simulink model "modelSimpleGenset"  (R2019a)
settings: Solver=FixedStepAuto  StartTime=0.0  StopTime=10.0  FixedStep=1e-1  RelTol=1e-3
model workspace (MAT data in the model file):
  avrDroop = 0.01
  avrKI = 10
  avrKP = 40
  governorDroop = 0.02
  inductiveInnerResistance = 0.48
  initialFieldVoltage = 0.676611722086
  maxFieldVoltage = 20
  minFieldVoltage = 0.01
  noLoadFrequency = 1.0101010101
  ratedPower = 9100000
  resistiveInnerResistance = 0.0019
values from neighbouring files (symbols this model uses):
  numberOfBuses = 2    [init.m]
libraries: simulink x8
settings Model: DataDictionary=dataGenerator.sldd  ParameterArgumentNames=ratedPower  OrderedModelArguments=off  Creator=michel.miyazaki  LastModifiedBy=thomas.evang
settings SimscapeCC: EditingMode=Restricted

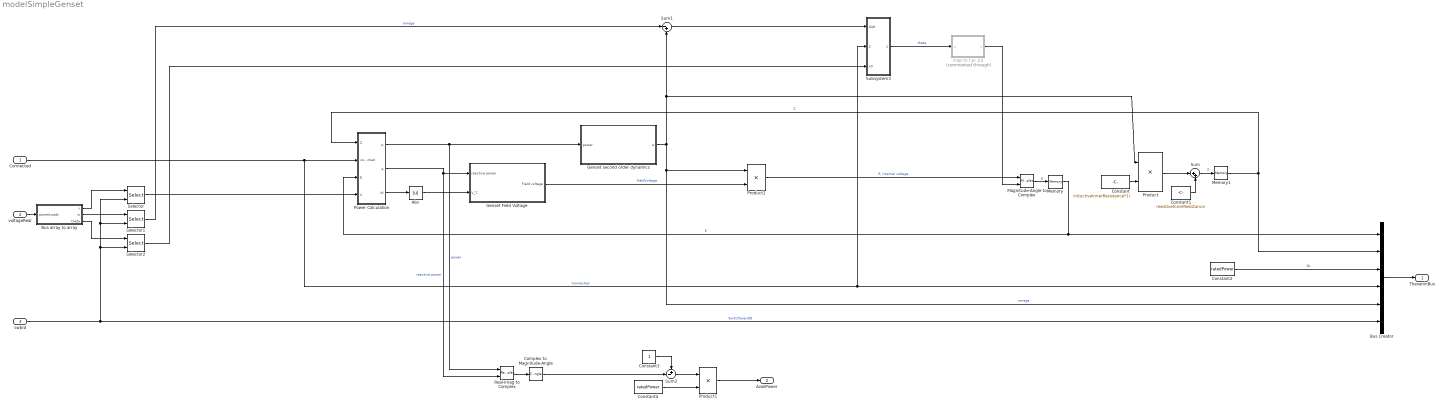
== system modelSimpleGenset ==
  Connected : Inport  OutDataTypeStr=boolean
  voltageReal : Inport  Port=2  OutDataTypeStr=Bus: swb  PortDimensions=[1 numberOfBuses]  Interpolate=off  BusOutputAsStruct=on
  swbId : Inport  Port=3
  Abs : Abs
  Bus Creator : BusCreator  Inputs=6  OutDataTypeStr=Bus: TheveninBus
  Bus array to array : Subsystem  TreatAsAtomicUnit=on
  Complex to Magnitude-Angle : ComplexToMagnitudeAngle  Output=Magnitude
  Constant : Constant  Value=inductiveInnerResistance*1i
  Constant1 : Constant  Value=resistiveInnerResistance
  Constant2 : Constant  Value=ratedPower
  Constant3 : Constant
  Constant4 : Constant  Value=ratedPower
  Genset Field Voltage : Subsystem
  Genset second order dynamics : Subsystem
  Magnitude-Angle to Complex : MagnitudeAngleToComplex
  Memory : Memory  InitialCondition=0.43*(1+1*1i)  LinearizeMemory=on  LinearizeAsDelay=on
  Memory1 : Memory  InitialCondition=resistiveInnerResistance+inductiveInnerResistance*1i*noLoadFrequency  LinearizeMemory=on  LinearizeAsDelay=on
  Power Calculation : Subsystem
  Product : Product
  Product1 : Product  Inputs=**  RndMeth=Zero
  Product2 : Product  Inputs=**  RndMeth=Zero
  Real-Imag to Complex : RealImagToComplex
  Selector : Selector  IndexOptions=Index vector (port)  Indices=[1 3]  OutputSizes=1
  Selector1 : Selector  IndexOptions=Index vector (port)  Indices=[1 3]  OutputSizes=1
  Selector2 : Selector  IndexOptions=Index vector (port)  Indices=[1 3]  OutputSizes=1
  Subsystem3 : Subsystem
  Sum : Sum  Inputs=|++
  Sum1 : Sum  Inputs=|-+
  Sum2 : Sum  Inputs=+-|
  "map to [-pi, pi]" : Subsystem  Commented=through
  TheveninBus : Outport  OutDataTypeStr=Bus: TheveninBus  BusOutputAsStruct=on
  AvailPower : Outport  Port=2  BusOutputAsStruct=on
  wires:
  Constant/1 -> Product/2
  Selector1/1 -> Sum1/1  "omega"
  Selector2/1 -> Subsystem3/3(x0)
  Product/1 -> Sum/1
  Constant1/1 -> Sum/2
  Sum/1 -> Memory1/1  "Z"
  Connected/1 -> Power Calculation/2(connected), Subsystem3/2(reset), Bus Creator/4  "Connected"
  Magnitude-Angle to Complex/1 -> Memory/1  "E"
  Sum1/1 -> Subsystem3/1(d/dt)
  Subsystem3/1(Out1) -> "map to [-pi, pi]"/1(u)  "theta"
  Product2/1 -> Magnitude-Angle to Complex/1  "E, internal voltage"
  Power Calculation/2(q) -> Real-Imag to Complex/2, Genset Field Voltage/1(reactive power)  "reactive power"
  Genset Field Voltage/1(Field voltage) -> Product2/2  "fieldVoltage"
  Power Calculation/1(p) -> Genset second order dynamics/1(power), Real-Imag to Complex/1  "power"
  Power Calculation/3(Vt) -> Abs/1
  Abs/1 -> Genset Field Voltage/2(V_T)
  Genset second order dynamics/1(w) -> Bus Creator/5, Product2/1, Product/1, Sum1/2  "omega"
  Memory1/1 -> Bus Creator/2, Power Calculation/1(Z)  "Z"
  Memory/1 -> Bus Creator/1, Power Calculation/3(E)  "E"
  "map to [-pi, pi]"/1(y) -> Magnitude-Angle to Complex/2
  Selector/1 -> Power Calculation/4(V)
  voltageReal/1 -> Bus array to array/1(powerLoads)
  Bus Creator/1 -> TheveninBus/1
  Constant2/1 -> Bus Creator/3  "Sb"
  swbId/1 -> Selector2/2, Selector1/2, Selector/2, Bus Creator/6  "SwitchboardID"
  Bus array to array/2(w) -> Selector1/1
  Bus array to array/3(theta) -> Selector2/1
  Bus array to array/1(v) -> Selector/1
  Sum2/1 -> Product1/1
  Real-Imag to Complex/1 -> Complex to Magnitude-Angle/1
  Constant4/1 -> Product1/2
  Complex to Magnitude-Angle/1 -> Sum2/2
  Constant3/1 -> Sum2/1
  Product1/1 -> AvailPower/1

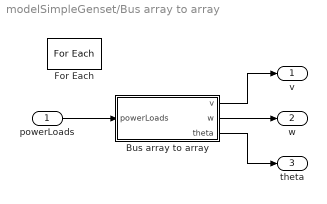
== system modelSimpleGenset/Bus array to array ==
  powerLoads : Inport  OutDataTypeStr=Bus: swb  Partition=on  PartitionDimension=1  PartitionWidth=1  PartitionOffset=0
  Bus array to array : Subsystem  TreatAsAtomicUnit=on
  For Each : ForEach  DisableCoverage=on  IndexMode=One-based
  v : Outport  ConcatenationDimension=1
  w : Outport  Port=2  ConcatenationDimension=1
  theta : Outport  Port=3  ConcatenationDimension=1
  wires:
  powerLoads/1 -> Bus array to array/1(powerLoads)
  Bus array to array/2(w) -> w/1
  Bus array to array/3(theta) -> theta/1
  Bus array to array/1(v) -> v/1

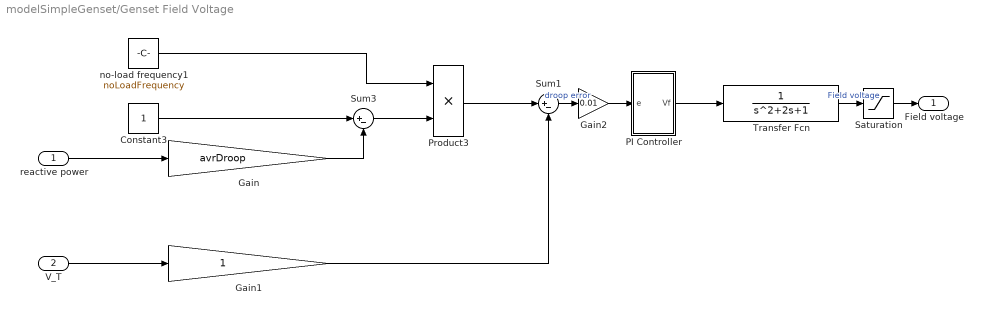
== system modelSimpleGenset/Genset Field Voltage ==
  reactive power : Inport
  V_T : Inport  Port=2
  Constant3 : Constant
  Gain : Gain  Gain=avrDroop
  Gain1 : Gain
  Gain2 : Gain  Gain=0.01
  PI Controller : Subsystem
  Product3 : Product  RndMeth=Zero
  Saturation : Saturate  UpperLimit=maxFieldVoltage  LowerLimit=minFieldVoltage  LinearizeAsGain=off  ZeroCross=off  OutMin=minFieldVoltage  OutMax=maxFieldVoltage  OutDataTypeStr=Inherit: Inherit via back propagation
  Sum1 : Sum  Inputs=|+-
  Sum3 : Sum  Inputs=|+-
  Transfer Fcn : TransferFcn
  no-load frequency1 : Constant  Value=noLoadFrequency
  Field voltage : Outport
  wires:
  Constant3/1 -> Sum3/1
  reactive power/1 -> Gain/1
  Gain/1 -> Sum3/2
  no-load frequency1/1 -> Product3/1
  Transfer Fcn/1 -> Saturation/1  "Field voltage"
  Sum3/1 -> Product3/2
  PI Controller/1(Vf) -> Transfer Fcn/1
  Product3/1 -> Sum1/1
  Sum1/1 -> Gain2/1  "droop error"
  V_T/1 -> Gain1/1
  Gain1/1 -> Sum1/2
  Saturation/1 -> Field voltage/1
  Gain2/1 -> PI Controller/1(e)

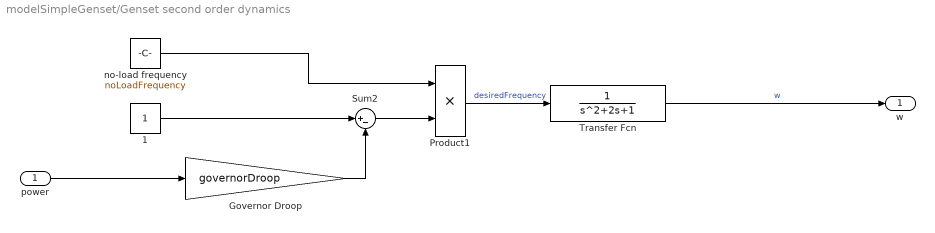
== system modelSimpleGenset/Genset second order dynamics ==
  power : Inport
  1 : Constant
  Governor Droop : Gain  Gain=governorDroop
  Product1 : Product  RndMeth=Zero
  Sum2 : Sum  Inputs=|+-
  Transfer Fcn : TransferFcn
  no-load frequency : Constant  Value=noLoadFrequency
  w : Outport
  wires:
  Transfer Fcn/1 -> w/1  "w"
  power/1 -> Governor Droop/1
  Governor Droop/1 -> Sum2/2
  1/1 -> Sum2/1
  Product1/1 -> Transfer Fcn/1  "desiredFrequency"
  no-load frequency/1 -> Product1/1
  Sum2/1 -> Product1/2

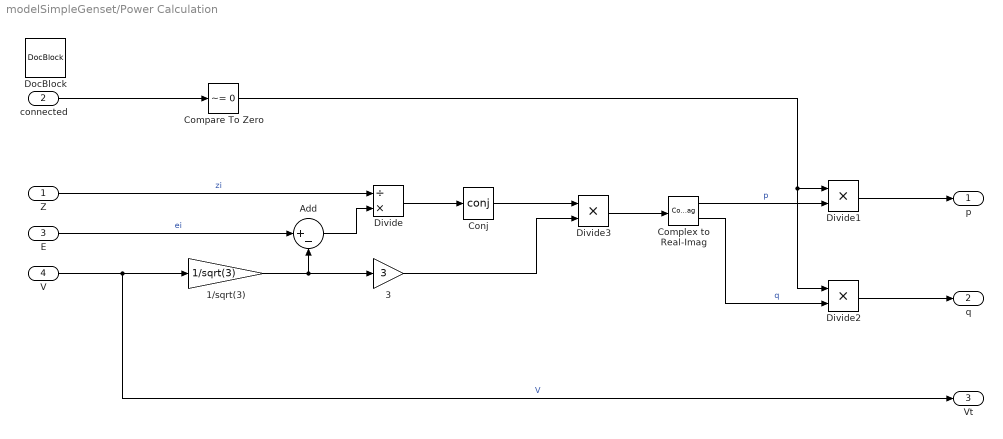
== system modelSimpleGenset/Power Calculation ==
  Z : Inport
  connected : Inport  Port=2
  E : Inport  Port=3
  V : Inport  Port=4
  1/sqrt(3) : Gain  Gain=1/sqrt(3)
  3 : Gain  Gain=3
  Add : Sum  Inputs=|+-
  Compare To Zero : simulink/Logic and Bit Operations/Compare To Zero  relop=~=  OutDataTypeStr=boolean
  Complex to Real-Imag : ComplexToRealImag
  Conj : Math  Operator=conj  SaturateOnIntegerOverflow=on
  Divide : Product  Inputs=/*
  Divide1 : Product
  Divide2 : Product
  Divide3 : Product  Inputs=**  OutDataTypeStr=double
  DocBlock : simulink/Model-Wide Utilities/DocBlock  DocumentType=Text
      content=|
      | function [p,q,Vt] = power(Z,connected,E,V)
      | %#codegen
      | if (connected)
      | Vt = V;
      | V = V/sqrt(3);
      | s = 3*V.*conj((E-V)./Z);
      | p = real(s);
      | q = imag(s);
      |
      | else
      | p = 0;
      | q = 0;
      | Vt =E*sqrt(3);
      | end
  p : Outport
  q : Outport  Port=2
  Vt : Outport  Port=3
  wires:
  connected/1 -> Compare To Zero/1
  Divide2/1 -> q/1
  Divide1/1 -> p/1
  E/1 -> Add/1  "ei"
  1/sqrt(3)/1 -> 3/1, Add/2
  Conj/1 -> Divide3/1
  Add/1 -> Divide/2
  Divide/1 -> Conj/1
  Z/1 -> Divide/1  "zi"
  Divide3/1 -> Complex to Real-Imag/1
  Complex to Real-Imag/1 -> Divide1/2  "p"
  Complex to Real-Imag/2 -> Divide2/2  "q"
  Compare To Zero/1 -> Divide1/1, Divide2/1
  V/1 -> Vt/1, 1/sqrt(3)/1  "V"
  3/1 -> Divide3/2

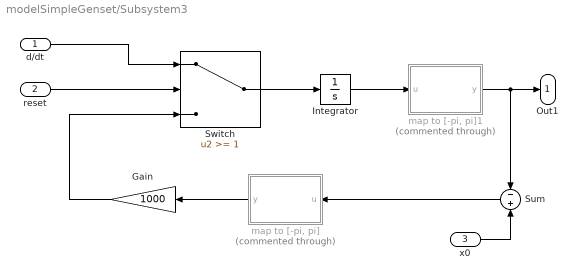
== system modelSimpleGenset/Subsystem3 ==
  d/dt : Inport
  reset : Inport  Port=2
  x0 : Inport  Port=3
  Gain : Gain  Gain=1000
  Integrator : Integrator  InitialCondition=pi/4  UpperSaturationLimit=pi  LowerSaturationLimit=0  WrapState=on  ZeroCross=off
  Sum : Sum  Inputs=-|+
  Switch : Switch  Threshold=1
  "map to [-pi, pi]" : Subsystem  Commented=through
  "map to [-pi, pi]1" : Subsystem  Commented=through
  Out1 : Outport
  wires:
  Sum/1 -> "map to [-pi, pi]"/1(u)
  d/dt/1 -> Switch/1
  reset/1 -> Switch/2
  "map to [-pi, pi]"/1(y) -> Gain/1
  Switch/1 -> Integrator/1
  x0/1 -> Sum/2
  Gain/1 -> Switch/3
  Integrator/1 -> "map to [-pi, pi]1"/1(u)
  "map to [-pi, pi]1"/1(y) -> Sum/1, Out1/1

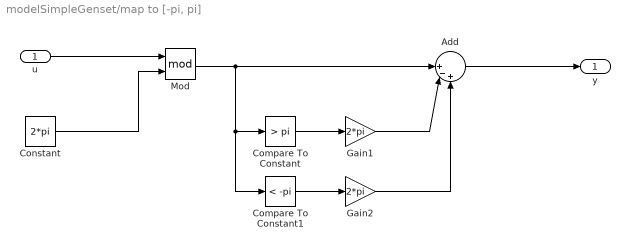
== system modelSimpleGenset/map to [-pi, pi] ==
  u : Inport
  Add : Sum  Inputs=||+-+
  Compare To Constant : simulink/Logic and Bit Operations/Compare To Constant  relop=>  const=pi  OutDataTypeStr=boolean
  Compare To Constant1 : simulink/Logic and Bit Operations/Compare To Constant  relop=<  const=-pi  OutDataTypeStr=boolean
  Constant : Constant  Value=2*pi
  Gain1 : Gain  Gain=2*pi
  Gain2 : Gain  Gain=2*pi
  Mod : Math  Operator=mod  SaturateOnIntegerOverflow=on
  y : Outport
  wires:
  Gain2/1 -> Add/3
  Constant/1 -> Mod/2
  Add/1 -> y/1
  Mod/1 -> Add/1, Compare To Constant1/1, Compare To Constant/1
  Gain1/1 -> Add/2
  u/1 -> Mod/1
  Compare To Constant/1 -> Gain1/1
  Compare To Constant1/1 -> Gain2/1

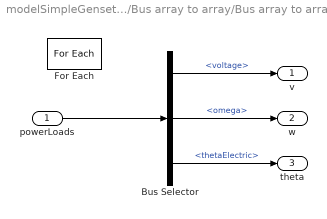
== system modelSimpleGenset/Bus array to array/Bus array to array ==
  powerLoads : Inport  OutDataTypeStr=Bus: swb  Partition=on  PartitionDimension=2  PartitionWidth=1  PartitionOffset=0
  Bus Selector : BusSelector  OutputSignals=voltage,omega,thetaElectric
  For Each : ForEach  DisableCoverage=on  IndexMode=One-based
  v : Outport  ConcatenationDimension=2
  w : Outport  Port=2  ConcatenationDimension=2
  theta : Outport  Port=3  ConcatenationDimension=2
  wires:
  powerLoads/1 -> Bus Selector/1
  Bus Selector/2 -> w/1  "<omega>"
  Bus Selector/3 -> theta/1  "<thetaElectric>"
  Bus Selector/1 -> v/1  "<voltage>"

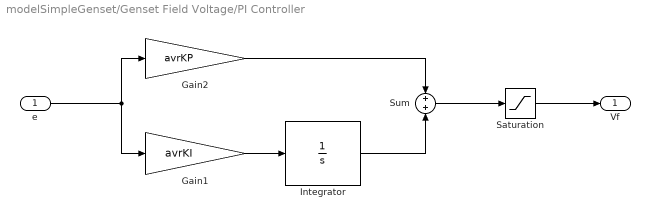
== system modelSimpleGenset/Genset Field Voltage/PI Controller ==
  e : Inport
  Gain1 : Gain  Gain=avrKI
  Gain2 : Gain  Gain=avrKP
  Integrator : Integrator  DisableCoverage=on  InitialCondition=initialFieldVoltage  LimitOutput=on  UpperSaturationLimit=maxFieldVoltage  LowerSaturationLimit=minFieldVoltage
  Saturation : Saturate  UpperLimit=maxFieldVoltage  LowerLimit=minFieldVoltage  LinearizeAsGain=off  ZeroCross=off  OutMin=minFieldVoltage  OutMax=maxFieldVoltage  OutDataTypeStr=Inherit: Inherit via back propagation
  Sum : Sum  Inputs=+|+
  Vf : Outport
  wires:
  Sum/1 -> Saturation/1
  e/1 -> Gain2/1, Gain1/1
  Saturation/1 -> Vf/1
  Integrator/1 -> Sum/2
  Gain2/1 -> Sum/1
  Gain1/1 -> Integrator/1

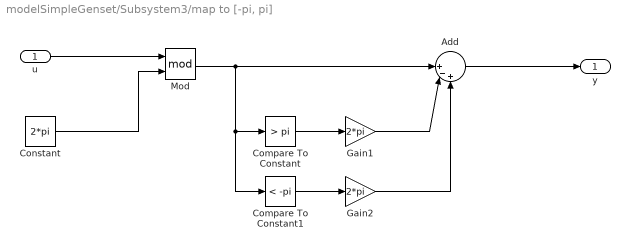
== system modelSimpleGenset/Subsystem3/map to [-pi, pi] ==
  u : Inport
  Add : Sum  Inputs=||+-+
  Compare To Constant : simulink/Logic and Bit Operations/Compare To Constant  relop=>  const=pi  OutDataTypeStr=boolean
  Compare To Constant1 : simulink/Logic and Bit Operations/Compare To Constant  relop=<  const=-pi  OutDataTypeStr=boolean
  Constant : Constant  Value=2*pi
  Gain1 : Gain  Gain=2*pi
  Gain2 : Gain  Gain=2*pi
  Mod : Math  Operator=mod  SaturateOnIntegerOverflow=on
  y : Outport
  wires:
  Gain2/1 -> Add/3
  Constant/1 -> Mod/2
  Add/1 -> y/1
  Mod/1 -> Add/1, Compare To Constant1/1, Compare To Constant/1
  Gain1/1 -> Add/2
  u/1 -> Mod/1
  Compare To Constant/1 -> Gain1/1
  Compare To Constant1/1 -> Gain2/1

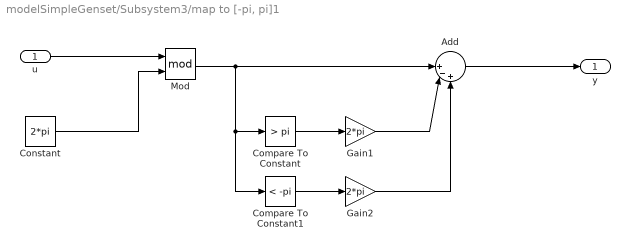
== system modelSimpleGenset/Subsystem3/map to [-pi, pi]1 ==
  u : Inport
  Add : Sum  Inputs=||+-+
  Compare To Constant : simulink/Logic and Bit Operations/Compare To Constant  relop=>  const=pi  OutDataTypeStr=boolean
  Compare To Constant1 : simulink/Logic and Bit Operations/Compare To Constant  relop=<  const=-pi  OutDataTypeStr=boolean
  Constant : Constant  Value=2*pi
  Gain1 : Gain  Gain=2*pi
  Gain2 : Gain  Gain=2*pi
  Mod : Math  Operator=mod  SaturateOnIntegerOverflow=on
  y : Outport
  wires:
  Compare To Constant1/1 -> Gain2/1
  Compare To Constant/1 -> Gain1/1
  u/1 -> Mod/1
  Gain1/1 -> Add/2
  Mod/1 -> Compare To Constant/1, Compare To Constant1/1, Add/1
  Add/1 -> y/1
  Constant/1 -> Mod/2
  Gain2/1 -> Add/3
